simulink model "BasciFiltering"  (R2020a)
settings: Solver=VariableStepAuto  StartTime=0.0  StopTime=20.0  RelTol=1e-3
libraries: dspsnks4 x1, dspvision x1, dspfdesign x1, dspsrcs4 x1
settings Model: Creator=Administrator  LastModifiedBy=Administrator

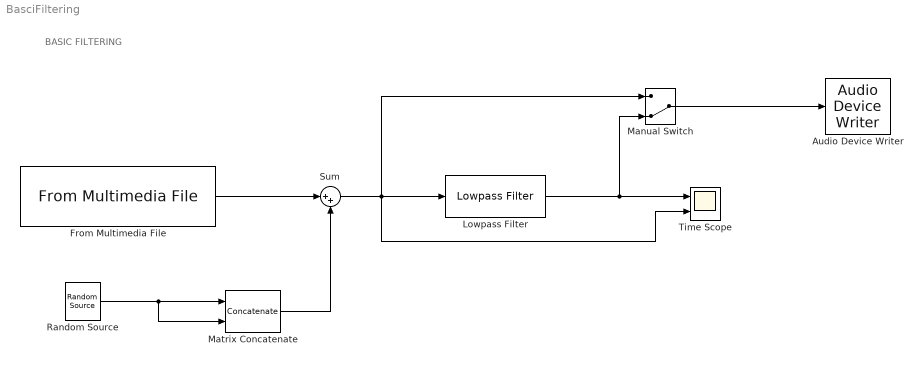
== system BasciFiltering ==
  note: BASIC FILTERING
  Audio Device Writer : dspsnks4/Audio Device Writer  Driver=DirectSound  Device=Default  InheritSampleRate=on  SampleRate=44100  BitDepth=16-bit integer  BufferSize=4096  NumBuffers=10  DefaultOutputChannelMapping=on  OutputChannelMapping=1:2  OutputNumUnderrunSamples=off  DriverIdx=1  DeviceWarnFlag=''
  From Multimedia File : dspvision/From Multimedia File  inputFilename=C:\Users\Administrator\Downloads\countdown-ten-seconds-76982.mp3  readRange=[1 Inf]  loop=on  numPlays=inf  outputStreams=Audio only  videoDataType=single  audioDataType=double  inheritSampleTime=on  userDefinedSampleTime=1/30  noAudioOutput=off  isIntensityVideo=off  fourcc=RGB  colorVideoFormat=Separate color signals  outputEOF=off  dataOrg=Column-major  audioFrameSize=1024  computeAudioFrameSize=off  outSamplingMode=Sample based
  Lowpass Filter : dspfdesign/Lowpass Filter  FilterType=FIR  DesignForMinimumOrder=on  FilterOrder=50  PassbandFrequency=9600  StopbandFrequency=10400  PassbandRipple=0.1  StopbandAttenuation=90  InheritSampleRate=off  SampleRate=44100  SimulateUsing=Interpreted execution  roundingMode=Floor  coeffsDataTypeStr=fixdt(1,16)
  Manual Switch : ManualSwitch  CurrentSetting=0
  Matrix Concatenate : Concatenate  Mode=Multidimensional array  ConcatenateDimension=2
  Random Source : dspsrcs4/Random Source  SrcType=Gaussian  NormMethod=Ziggurat  CltLength=12  MinVal=0  MaxVal=1  MeanVal=0  VarVal=0.001  RepMode=Repeatable  rawSeed=1  IsInherit=off  SampMode=Discrete  SampTime=1/24000  SampFrame=1024  DataType=Double  OutComplex=Real  OutputFrames=off
  Sum : Sum  Inputs=|++
  Time Scope : Scope  NumInputPorts=2
  wires:
  Sum/1 -> Time Scope/2, Manual Switch/1, Lowpass Filter/1
  Lowpass Filter/1 -> Manual Switch/2, Time Scope/1
  Manual Switch/1 -> Audio Device Writer/1
  From Multimedia File/1 -> Sum/1
  Matrix Concatenate/1 -> Sum/2
  Random Source/1 -> Matrix Concatenate/2, Matrix Concatenate/1
